simulink model "controllerReference_r2019a"  (R2019a)
settings: Solver=ode23tb  StartTime=0.0  StopTime=Inf  FixedStep=.05  RelTol=1e-3  EnableMultiTasking=on
StartFcn:
  | %tic
StopFcn:
  | %toc
model workspace (MAT data in the model file):
  A_mu = 10
  B_reff = 8.386
  Cz = 7766.25
  DCT_Param : struct (value not decoded)
  DLCXref = [0 6 7 14 33.5 34 42 50 60]
  DLCYref = [0 0 -4.5 -4 -3.75 1.5 0.5 0 0]
  D_reff = 0.25826
  Downshift_Speeds = [9.5625 12.9375 16.3125 19.6875 23.0625 26.4375 29.8125 33.1875 36.5625 39.9375 43.3125 46.6875 ... (28 elements, 4x7)]
  EngRevLim = 7000
  Pedal_Positions = [0.1 0.4 0.5 0.9]
  SUS : struct (value not decoded)
  Upshift_Speeds = [12.9375 16.3125 19.6875 33 26.4375 29.8125 33.1875 52.5 39.9375 43.3125 46.6875 77.25 ... (28 elements, 4x7)]
  VEH : struct (value not decoded)
  V_o = 16.7
  V_xlow = 1
  WH : struct (value not decoded)
  a = 1.4
  alpha_max = 1.5
  alpha_min = -1.5
  b = 1.8
  c_zo = 209651
  epsilon = 0.1
  h = 0.134
  path : struct (value not decoded)
  pio = 220000
  q_Fcx = 0
  q_Fz2 = 15.4
  q_Fzy = 0
  q_reo = 0.9974
  q_sx1 = -0.007764
  q_sx10 = 0.2824
  q_sx11 = 5.349
  q_sx12 = 0
  q_sx13 = 0
  q_sx14 = 0
  q_sx2 = 1.1915
  q_sx3 = 0.013948
  q_sx4 = 4.912
  q_sx5 = 1.02
  q_sx6 = 22.83
  q_sx7 = 0.7104
  q_sx8 = -0.023393
  q_sx9 = 0.6581
  q_sy1 = 0.00702
  q_sy2 = 0
  q_sy3 = 0.001515
  q_sy4 = 8.514e-05
  q_sy5 = 0
  q_sy6 = 0
  q_sy7 = 0.9008
  q_sy8 = -0.4089
  q_v1 = 0.0007742
  q_v2 = 0.04667
  r_Bx1 = 12.531
  r_Bx2 = 9.532
  r_Bx3 = 0
  r_By1 = 10.615
  r_By2 = 7.705
  r_By3 = 3.433e-06
  r_By4 = 0
  r_Cx1 = 1.019
  r_Cy1 = 1.0585
  r_Ex1 = -0.4487
  r_Ex2 = -0.4726
  r_Ey1 = 0.3132
  r_Ey2 = 7.63e-06
  r_Hx1 = 0.0002374
  r_Hy1 = 0.011646
  r_Hy2 = 7.63e-06
  r_Vy1 = 0.05654
  r_Vy2 = 7.63e-06
  r_Vy3 = 0
  r_Vy4 = 99.9
  r_Vy5 = 2
  r_Vy6 = 15.814
  r_o = 0.3135
  vehWidth = 2
  w = 1
symbols that are objects in the model workspace (value not decoded): VEH
undefined symbols (not defined in the file): curvature, curvatures, pathPoints, speedProfile, splineParams, Steer, Ts, velocities, xDotRef, xRef, yDotRef, yRef
libraries: autolibutils x5, simulink x5, sim3dlib x4, mpcadaslib x1, autolibshared x1, vrlib x1, vehdynlibviscommon x1
(part 2 of 2)

== system controllerReference_r2019a/Environment/Ground Feedback/3D Engine ==
  Friction : Inport
  Bus Creator : BusCreator  Inputs=4
  Bus Creator2 : BusCreator  Inputs=4
  Bus Creator3 : BusCreator  Inputs=2
  Bus Selector : BusSelector  OutputSignals=HitLoc
  Data Type Conversion : DataTypeConversion
  Demux : Demux
  Demux1 : Demux
  Passenger Vehicle Ray Trace Set : sim3dlib/Vehicle Terrain Sensor  ActorTag=SimulinkVehicle1  VehExtEn=Constant  TireRadiiExt=Constant  VehCntrLngthVal=0  TireRadiiVal=0  VehRayLngth=10  LfRayLngth=20  RfRayLngth=20  LrRayLngth=20  RrRayLngth=20  VehRayOffset=0  LfRayOffset=-1  RfRayOffset=-1  LrRayOffset=-1  RrRayOffset=-1  VehEn=on  LfEn=on  RfEn=on  LrEn=on  RrEn=on  DbgEn=off  Ts=.03  aMode=2
      settings: SourceProductName=Vehicle Dynamics Blockset  SourceProductBaseCode=VE
  Rate Transition : RateTransition
  Reshape10 : Reshape  OutputDimensionality=Row vector (2-D)
  Selector1 : Selector  InputPortWidth=5  IndexOptions=Index vector (dialog)  Indices=[2:5]  OutputSizes=1
  Signal Specification : SignalSpecification  Unit=m
  Signal Specification1 : SignalSpecification  Unit=1
  Terminator1 : Terminator
  Terminator2 : Terminator
  Zend Select : Selector  NumberOfDimensions=2  InputPortWidth=3  IndexOptions=Select all,Index vector (dialog)  Indices=[1 3],3  OutputSizes=1,1
  Ground : Outport
  wires:
  Selector1/1 -> Rate Transition/1
  Zend Select/1 -> Reshape10/1
  Bus Selector/1 -> Zend Select/1  "<HitLoc>"
  Passenger Vehicle Ray Trace Set/2 -> Terminator1/1
  Passenger Vehicle Ray Trace Set/3 -> Terminator2/1
  Reshape10/1 -> Selector1/1
  Passenger Vehicle Ray Trace Set/1 -> Bus Selector/1
  Rate Transition/1 -> Data Type Conversion/1
  Demux/2 -> Bus Creator/2  "G_FR_z"
  Demux/1 -> Bus Creator/1  "G_FL_z"
  Demux/4 -> Bus Creator/4  "G_RR_z"
  Demux/3 -> Bus Creator/3  "G_RL_z"
  Signal Specification/1 -> Demux/1
  Signal Specification1/1 -> Demux1/1
  Demux1/1 -> Bus Creator2/1  "mu_FL"
  Bus Creator/1 -> Bus Creator3/1  "z"
  Demux1/3 -> Bus Creator2/3  "mu_RL"
  Demux1/4 -> Bus Creator2/4  "mu_RR"
  Demux1/2 -> Bus Creator2/2  "mu_FR"
  Bus Creator2/1 -> Bus Creator3/2  "mu"
  Bus Creator3/1 -> Ground/1
  Friction/1 -> Signal Specification1/1
  Data Type Conversion/1 -> Signal Specification/1

== system controllerReference_r2019a/Environment/Ground Feedback/Constant ==
  Friction : Inport
  Bus Creator : BusCreator  Inputs=4
  Bus Creator2 : BusCreator  Inputs=4
  Bus Creator3 : BusCreator  Inputs=2
  Constant1 : Constant  Value=zeros(4,1)
  Demux : Demux
  Demux1 : Demux
  Signal Specification : SignalSpecification  Unit=m
  Signal Specification1 : SignalSpecification  Unit=1
  Ground : Outport
  wires:
  Constant1/1 -> Signal Specification/1
  Signal Specification/1 -> Demux/1
  Demux/4 -> Bus Creator/4  "G_RR_z"
  Demux/1 -> Bus Creator/1  "G_FL_z"
  Demux/3 -> Bus Creator/3  "G_RL_z"
  Demux/2 -> Bus Creator/2  "G_FR_z"
  Bus Creator/1 -> Bus Creator3/1  "z"
  Demux1/3 -> Bus Creator2/3  "mu_RL"
  Demux1/4 -> Bus Creator2/4  "mu_RR"
  Demux1/1 -> Bus Creator2/1  "mu_FL"
  Demux1/2 -> Bus Creator2/2  "mu_FR"
  Bus Creator2/1 -> Bus Creator3/2  "mu"
  Friction/1 -> Signal Specification1/1
  Signal Specification1/1 -> Demux1/1
  Bus Creator3/1 -> Ground/1

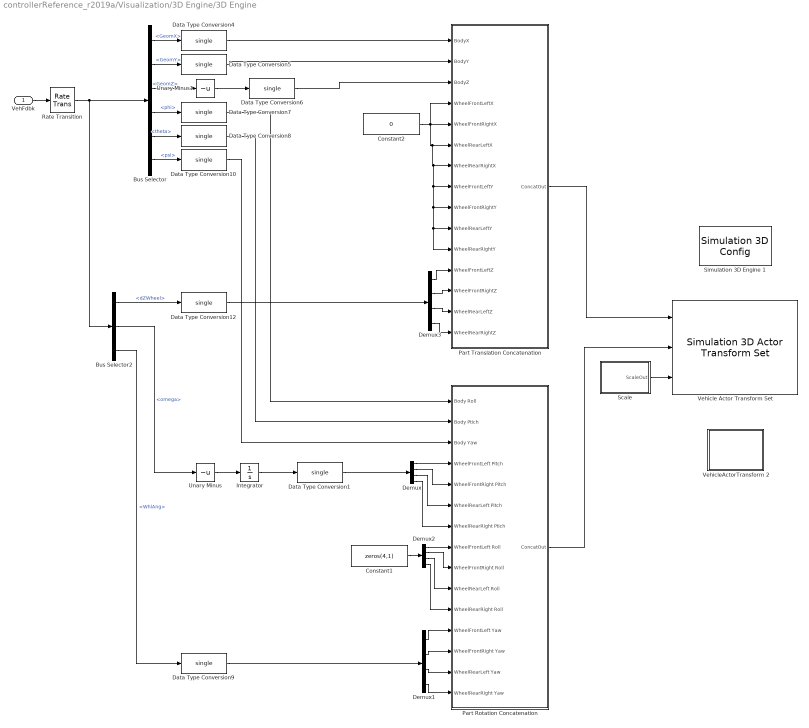
== system controllerReference_r2019a/Visualization/3D Engine/3D Engine ==
  VehFdbk : Inport
  Bus Selector : BusSelector  OutputSignals=Body.GeomX,Body.GeomY,Body.GeomZ,Body.phi,Body.theta,Body.psi
  Bus Selector2 : BusSelector  OutputSignals=Wheels.dZWheel,Wheels.omega,Driveline.WhlAng
  Constant1 : Constant  Value=zeros(4,1)  OutDataTypeStr=single
  Constant2 : Constant  Value=0  OutDataTypeStr=single
  Data Type Conversion{1,4..10,12} (9 alike) : DataTypeConversion  OutDataTypeStr=single
  Demux{,1..3} (4 alike) : Demux
  Integrator : Integrator  WrapState=on  WrappedStateUpperValue=2*pi  WrappedStateLowerValue=0  ZeroCross=off
  Part Rotation Concatenation : Subsystem
  Part Translation Concatenation : Subsystem
  Rate Transition : RateTransition  OutPortSampleTime=dt3D
  Scale : Subsystem
  Simulation 3D Engine 1 : sim3dlib/Simulation 3D Config  Priority=1  ProjectFormat=Executable  ProjectName=VehicleSimulation.exe  SceneDesc=Double lane change  OpVisEn=off  Ts=dt3D  aMode=2
      settings: AttributesFormatString=Priority: %<Priority>  SourceProductName=Vehicle Dynamics Blockset  SourceProductBaseCode=VE
  Unary Minus : UnaryMinus
  Unary Minus1 : UnaryMinus
  Vehicle Actor Transform Set : sim3dlib/Simulation 3D Actor Transform Set  ActorTag=SimulinkVehicle1  ActorType=Passenger vehicle  PassVehMesh=Muscle car  VehColor=Red  NumberOfParts=5  CustNumOfParts=3  Translation=[VEH.InitialLongPosition VEH.InitialLatPosition -VEH.InitialVertPosition; 0 0 0; 0 0 0; 0 0 0; 0 0 0]  Rotation=[VEH.InitialRollAngle VEH.InitialPitchAngle VEH.InitialYawAngle; 0 0 0; 0 0 0; 0 0 0; 0 0 0]  Scale=[1 1 1; 1 1 1; 1 1 1; 1 1 1; 1 1 1]  Ts=dt3D  aMode=2
      settings: SourceProductName=Vehicle Dynamics Blockset  SourceProductBaseCode=VE
  VehicleActorTransform 2 : Subsystem  mask{depth=-5}
      mask prompts: depth "Initital Z position, depth (m):"
  wires:
  Unary Minus1/1 -> Data Type Conversion6/1
  Unary Minus/1 -> Integrator/1
  Bus Selector2/1 -> Data Type Conversion12/1  "<dZWheel>"
  Rate Transition/1 -> Bus Selector/1, Bus Selector2/1
  Scale/1(ScaleOut) -> Vehicle Actor Transform Set/3
  Demux/4 -> Part Rotation Concatenation/7(WheelRearRight Ptich)
  Demux/3 -> Part Rotation Concatenation/6(WheelRearLeft Pitch)
  Demux/2 -> Part Rotation Concatenation/5(WheelFrontRight Pitch)
  Demux/1 -> Part Rotation Concatenation/4(WheelFrontLeft Pitch)
  Constant1/1 -> Demux2/1
  Bus Selector/4 -> Data Type Conversion7/1  "<phi>"
  Part Rotation Concatenation/1(ConcatOut) -> Vehicle Actor Transform Set/2
  Part Translation Concatenation/1(ConcatOut) -> Vehicle Actor Transform Set/1
  Data Type Conversion12/1 -> Demux3/1
  Demux3/4 -> Part Translation Concatenation/15(WheelRearRightZ)
  Demux3/3 -> Part Translation Concatenation/14(WheelRearLeftZ)
  Demux3/1 -> Part Translation Concatenation/12(WheelFrontLeftZ)
  Demux3/2 -> Part Translation Concatenation/13(WheelFrontRightZ)
  VehFdbk/1 -> Rate Transition/1
  Data Type Conversion6/1 -> Part Translation Concatenation/3(BodyZ)
  Demux1/4 -> Part Rotation Concatenation/15(WheelRearRight Yaw)
  Demux1/3 -> Part Rotation Concatenation/14(WheelRearLeft Yaw)
  Demux2/1 -> Part Rotation Concatenation/8(WheelFrontLeft Roll)
  Demux2/2 -> Part Rotation Concatenation/9(WheelFrontRight Roll)
  Demux2/3 -> Part Rotation Concatenation/10(WheelRearLeft Roll)
  Demux2/4 -> Part Rotation Concatenation/11(WheelRearRight Roll)
  Bus Selector2/3 -> Data Type Conversion9/1  "<WhlAng>"
  Bus Selector2/2 -> Unary Minus/1  "<omega>"
  Data Type Conversion9/1 -> Demux1/1
  Demux1/1 -> Part Rotation Concatenation/12(WheelFrontLeft Yaw)
  Demux1/2 -> Part Rotation Concatenation/13(WheelFrontRight Yaw)
  Integrator/1 -> Data Type Conversion1/1
  Data Type Conversion1/1 -> Demux/1
  Data Type Conversion8/1 -> Part Rotation Concatenation/2(Body Ptich)
  Data Type Conversion5/1 -> Part Translation Concatenation/2(BodyY)
  Data Type Conversion10/1 -> Part Rotation Concatenation/3(Body Yaw)
  Constant2/1 -> Part Translation Concatenation/5(WheelFrontRightX), Part Translation Concatenation/6(WheelRearLeftX), Part Translation Concatenation/7(WheelRearRightX), Part Translation Concatenation/8(WheelFrontLeftY), Part Translation Concatenation/9(WheelFrontRightY), Part Translation Concatenation/10(WheelRearLeftY), Part Translation Concatenation/11(WheelRearRightY), Part Translation Concatenation/4(WheelFrontLeftX)
  Data Type Conversion4/1 -> Part Translation Concatenation/1(BodyX)
  Data Type Conversion7/1 -> Part Rotation Concatenation/1(Body Roll)
  Bus Selector/1 -> Data Type Conversion4/1  "<GeomX>"
  Bus Selector/2 -> Data Type Conversion5/1  "<GeomY>"
  Bus Selector/3 -> Unary Minus1/1  "<GeomZ>"
  Bus Selector/6 -> Data Type Conversion10/1  "<psi>"
  Bus Selector/5 -> Data Type Conversion8/1  "<theta>"

== system controllerReference_r2019a/Visualization/3D Engine/3D Engine Disabled ==
  VehFdbk : Inport
  Terminator : Terminator
  wires:
  VehFdbk/1 -> Terminator/1

== system controllerReference_r2019a/Visualization/ISO 15037-1:2006/Disabled ==
  VehFdbk : Inport
  Cntrl : Inport  Port=2
  Terminator : Terminator
  Terminator1 : Terminator
  wires:
  Cntrl/1 -> Terminator/1
  VehFdbk/1 -> Terminator1/1

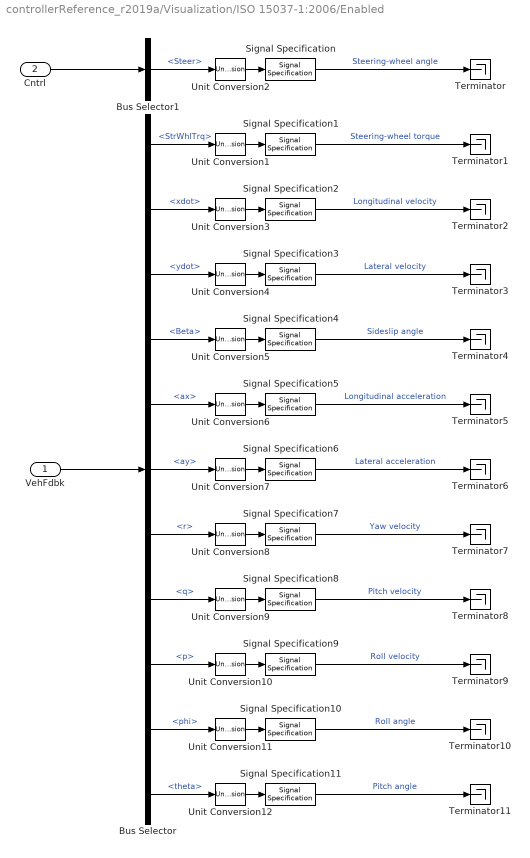
== system controllerReference_r2019a/Visualization/ISO 15037-1:2006/Enabled ==
  VehFdbk : Inport
  Cntrl : Inport  Port=2
  Bus Selector : BusSelector  OutputSignals=Steering.StrWhlTrq,Body.xdot,Body.ydot,Body.Beta,Body.ax,Body.ay,Body.r,Body.q,Body.p,Body.phi,Body.theta
  Bus Selector1 : BusSelector  OutputSignals=Steer
  Signal Specification{,4,10..11} (4 alike) : SignalSpecification  Unit=deg
  Signal Specification1 : SignalSpecification  Unit=N*m
  Signal Specification2 : SignalSpecification  Unit=km/h
  Signal Specification3 : SignalSpecification  Unit=m/s
  Signal Specification5 : SignalSpecification  Unit=m/s^2
  Signal Specification6 : SignalSpecification  Unit=m/s^2
  Signal Specification7 : SignalSpecification  Unit=deg/s
  Signal Specification8 : SignalSpecification  Unit=deg/s
  Signal Specification9 : SignalSpecification  Unit=deg/s
  Terminator{,1..11} (12 alike) : Terminator
  Unit Conversion{1..12} (12 alike) : UnitConversion
  wires:
  Bus Selector/11 -> Unit Conversion12/1  "<theta>"
  Signal Specification11/1 -> Terminator11/1  "Pitch angle"
  Unit Conversion12/1 -> Signal Specification11/1
  Bus Selector/10 -> Unit Conversion11/1  "<phi>"
  Unit Conversion11/1 -> Signal Specification10/1
  Signal Specification10/1 -> Terminator10/1  "Roll angle"
  Bus Selector/9 -> Unit Conversion10/1  "<p>"
  Signal Specification9/1 -> Terminator9/1  "Roll velocity"
  Unit Conversion10/1 -> Signal Specification9/1
  Bus Selector/8 -> Unit Conversion9/1  "<q>"
  Unit Conversion9/1 -> Signal Specification8/1
  Signal Specification8/1 -> Terminator8/1  "Pitch velocity"
  Bus Selector/7 -> Unit Conversion8/1  "<r>"
  Signal Specification7/1 -> Terminator7/1  "Yaw velocity"
  Unit Conversion8/1 -> Signal Specification7/1
  Bus Selector/6 -> Unit Conversion7/1  "<ay>"
  Unit Conversion7/1 -> Signal Specification6/1
  Signal Specification6/1 -> Terminator6/1  "Lateral acceleration"
  Bus Selector/5 -> Unit Conversion6/1  "<ax>"
  Signal Specification5/1 -> Terminator5/1  "Longitudinal acceleration"
  Unit Conversion6/1 -> Signal Specification5/1
  Bus Selector/4 -> Unit Conversion5/1  "<Beta>"
  Unit Conversion5/1 -> Signal Specification4/1
  Signal Specification4/1 -> Terminator4/1  "Sideslip angle"
  Bus Selector/3 -> Unit Conversion4/1  "<ydot>"
  Signal Specification3/1 -> Terminator3/1  "Lateral velocity"
  Unit Conversion4/1 -> Signal Specification3/1
  Bus Selector/2 -> Unit Conversion3/1  "<xdot>"
  Unit Conversion3/1 -> Signal Specification2/1
  Signal Specification2/1 -> Terminator2/1  "Longitudinal velocity"
  Signal Specification1/1 -> Terminator1/1  "Steering-wheel torque"
  Unit Conversion1/1 -> Signal Specification1/1
  Bus Selector/1 -> Unit Conversion1/1  "<StrWhlTrq>"
  Signal Specification/1 -> Terminator/1  "Steering-wheel angle"
  Unit Conversion2/1 -> Signal Specification/1
  Bus Selector1/1 -> Unit Conversion2/1  "<Steer>"
  Cntrl/1 -> Bus Selector1/1
  VehFdbk/1 -> Bus Selector/1

== system controllerReference_r2019a/Controllers/Brake Controller/Brake Pressure Control/Bang Bang ABS ==
  Pref : Inport
  xdot : Inport  Port=2
  <Kappa> : Inport  Port=3
  Abs : Abs
  Add : Sum  Inputs=-+
  Bang-bang controller : Subsystem  mask(Sign){}
      mask help: y = sign(x)
      mask Help: Sign Function:\n\t\t\ty = 1 if x > 0\n\t\t\ty = 0 if x = 0\n\t\t\ty = -1 if x < 0
      mask Display: plot(-50,-50,50,50,[-50,50],[0,0],[0,0],[-50,50],[-40,0],[-30,-30],[0,40],[30,30])
  Compare To Constant : simulink/Logic and Bit Operations/Compare To Constant  relop=>=  const=.2  OutDataTypeStr=boolean
  Compare To Constant1 : simulink/Logic and Bit Operations/Compare To Constant  relop=>=  const=.75  OutDataTypeStr=boolean
  Compare To Constant2 : simulink/Logic and Bit Operations/Compare To Constant  relop=>=  const=.5  OutDataTypeStr=boolean
  Constant : Constant  Value=.25
  Debounce : autolibutils/Debounce  DbcOn_Cnts=.1*.001  DbcOff_Cnts=.1*.001  aMode=aMode
      settings: SourceProductName=Powertrain Blockset  SourceProductBaseCode=PW
  Gain : Gain  Gain=200
  Logical Operator : Logic  Inputs=3  AllPortsSameDT=off  OutDataTypeStr=boolean
  Rate Transition : RateTransition  Deterministic=off  OutPortSampleTime=.001
  Rate Transition1 : RateTransition  Deterministic=off
  Switch : Switch  Criteria=u2 > Threshold  ZeroCross=off
  PCmd : Outport
  wires:
  Bang-bang controller/1(out_1) -> Gain/1
  Add/1 -> Bang-bang controller/1(in_1)
  Rate Transition1/1 -> PCmd/1
  <Kappa>/1 -> Rate Transition/1
  Pref/1 -> Switch/3, Compare To Constant1/1  "Pref"
  Constant/1 -> Add/2  "slip ref"
  Switch/1 -> Rate Transition1/1
  Rate Transition/1 -> Add/1, Compare To Constant/1
  Logical Operator/1 -> Debounce/1
  Compare To Constant/1 -> Logical Operator/2
  Compare To Constant1/1 -> Logical Operator/3
  Debounce/1 -> Switch/2
  xdot/1 -> Abs/1
  Abs/1 -> Compare To Constant2/1
  Compare To Constant2/1 -> Logical Operator/1
  Gain/1 -> Switch/1

== system controllerReference_r2019a/Controllers/Brake Controller/Brake Pressure Control/Open Loop ==
  Pref : Inport
  PCmd : Outport
  wires:
  Pref/1 -> PCmd/1  "Reference Slip"

== system controllerReference_r2019a/Controllers/Transmission Controller/Transmission Controller/TCM ==
  AccCmd : Inport
  EngSpd : Inport  Port=2
  VehSpdFdbk : Inport  Port=3
  function : TriggerPort  TriggerType=function-call  VariantControl=Variant
  Neutral Select : Subsystem
  Prop Shaft Speed LPF : DiscreteTransferFcn  Numerator=[0.000000000000000 0.009950166250832 ]  Denominator=[1.000000000000000 -0.990049833749168 ]  mask(DiscretizedDiscreteTransferFcn){}
      mask init:
      | %zoh
  TCM Shift Controller : Stateflow chart  TreatAsAtomicUnit=on
  prop speed to vehicle speed : Gain  Gain=0.45
  Gear Select : Outport
  wires:
  VehSpdFdbk/1 -> Prop Shaft Speed LPF/1
  TCM Shift Controller/1(GearState) -> Gear Select/1  "GearCmd"
  AccCmd/1 -> Neutral Select/1(AccCmd), TCM Shift Controller/2(pedal)  "AccCmd"
  Neutral Select/1(Neutral Select) -> TCM Shift Controller/3(Neutral)
  EngSpd/1 -> Neutral Select/2(EngSpd)
  prop speed to vehicle speed/1 -> TCM Shift Controller/1(speed)
  Prop Shaft Speed LPF/1 -> prop speed to vehicle speed/1

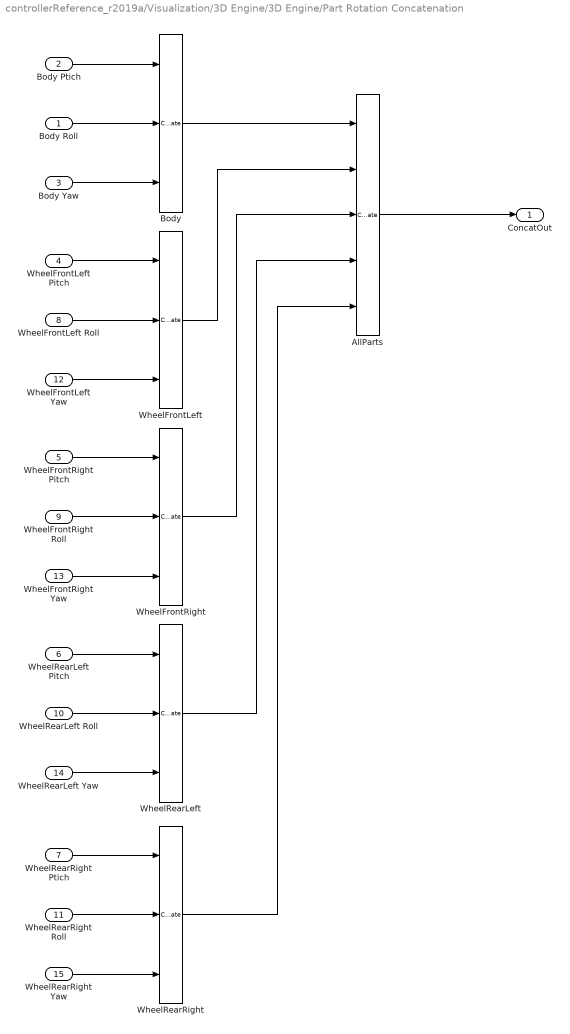
== system controllerReference_r2019a/Visualization/3D Engine/3D Engine/Part Rotation Concatenation ==
  Body Roll : Inport
  Body Ptich : Inport  Port=2
  Body Yaw : Inport  Port=3
  WheelFrontLeft Pitch : Inport  Port=4
  WheelFrontRight Pitch : Inport  Port=5
  WheelRearLeft Pitch : Inport  Port=6
  WheelRearRight Ptich : Inport  Port=7
  WheelFrontLeft Roll : Inport  Port=8
  WheelFrontRight Roll : Inport  Port=9
  WheelRearLeft Roll : Inport  Port=10
  WheelRearRight Roll : Inport  Port=11
  WheelFrontLeft Yaw : Inport  Port=12
  WheelFrontRight Yaw : Inport  Port=13
  WheelRearLeft Yaw : Inport  Port=14
  WheelRearRight Yaw : Inport  Port=15
  AllParts : Concatenate  NumInputs=5  Mode=Multidimensional array
  Body : Concatenate  NumInputs=3  Mode=Multidimensional array  ConcatenateDimension=2
  WheelFrontLeft : Concatenate  NumInputs=3  Mode=Multidimensional array  ConcatenateDimension=2
  WheelFrontRight : Concatenate  NumInputs=3  Mode=Multidimensional array  ConcatenateDimension=2
  WheelRearLeft : Concatenate  NumInputs=3  Mode=Multidimensional array  ConcatenateDimension=2
  WheelRearRight : Concatenate  NumInputs=3  Mode=Multidimensional array  ConcatenateDimension=2
  ConcatOut : Outport
  wires:
  Body Ptich/1 -> Body/1
  Body Yaw/1 -> Body/3
  WheelFrontLeft Pitch/1 -> WheelFrontLeft/1
  WheelFrontLeft Yaw/1 -> WheelFrontLeft/3
  WheelFrontLeft Roll/1 -> WheelFrontLeft/2
  Body Roll/1 -> Body/2
  WheelFrontLeft/1 -> AllParts/2
  WheelRearRight Ptich/1 -> WheelRearRight/1
  Body/1 -> AllParts/1
  WheelRearLeft/1 -> AllParts/4
  WheelFrontRight/1 -> AllParts/3
  WheelRearRight Yaw/1 -> WheelRearRight/3
  WheelFrontRight Roll/1 -> WheelFrontRight/2
  WheelFrontRight Pitch/1 -> WheelFrontRight/1
  WheelRearRight Roll/1 -> WheelRearRight/2
  WheelRearLeft Yaw/1 -> WheelRearLeft/3
  AllParts/1 -> ConcatOut/1
  WheelRearLeft Roll/1 -> WheelRearLeft/2
  WheelRearRight/1 -> AllParts/5
  WheelRearLeft Pitch/1 -> WheelRearLeft/1
  WheelFrontRight Yaw/1 -> WheelFrontRight/3

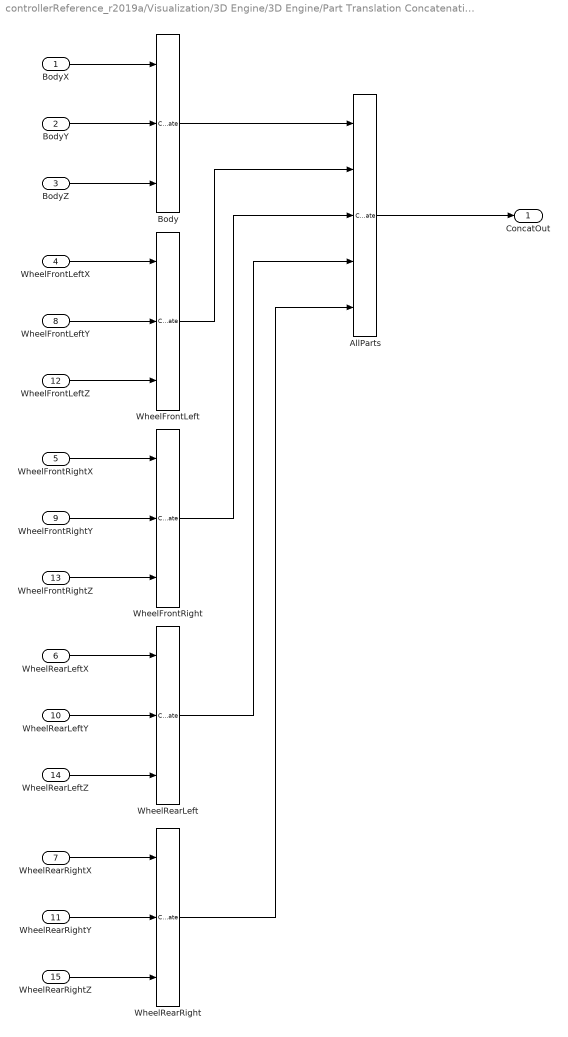
== system controllerReference_r2019a/Visualization/3D Engine/3D Engine/Part Translation Concatenation ==
  BodyX : Inport
  BodyY : Inport  Port=2
  BodyZ : Inport  Port=3
  WheelFrontLeftX : Inport  Port=4
  WheelFrontRightX : Inport  Port=5
  WheelRearLeftX : Inport  Port=6
  WheelRearRightX : Inport  Port=7
  WheelFrontLeftY : Inport  Port=8
  WheelFrontRightY : Inport  Port=9
  WheelRearLeftY : Inport  Port=10
  WheelRearRightY : Inport  Port=11
  WheelFrontLeftZ : Inport  Port=12
  WheelFrontRightZ : Inport  Port=13
  WheelRearLeftZ : Inport  Port=14
  WheelRearRightZ : Inport  Port=15
  AllParts : Concatenate  NumInputs=5  Mode=Multidimensional array
  Body : Concatenate  NumInputs=3  Mode=Multidimensional array  ConcatenateDimension=2
  WheelFrontLeft : Concatenate  NumInputs=3  Mode=Multidimensional array  ConcatenateDimension=2
  WheelFrontRight : Concatenate  NumInputs=3  Mode=Multidimensional array  ConcatenateDimension=2
  WheelRearLeft : Concatenate  NumInputs=3  Mode=Multidimensional array  ConcatenateDimension=2
  WheelRearRight : Concatenate  NumInputs=3  Mode=Multidimensional array  ConcatenateDimension=2
  ConcatOut : Outport
  wires:
  BodyX/1 -> Body/1
  BodyZ/1 -> Body/3
  WheelFrontLeftX/1 -> WheelFrontLeft/1
  WheelFrontLeftZ/1 -> WheelFrontLeft/3
  WheelFrontLeftY/1 -> WheelFrontLeft/2
  BodyY/1 -> Body/2
  WheelFrontLeft/1 -> AllParts/2
  WheelRearRightX/1 -> WheelRearRight/1
  Body/1 -> AllParts/1
  WheelRearLeft/1 -> AllParts/4
  WheelFrontRight/1 -> AllParts/3
  WheelRearRightZ/1 -> WheelRearRight/3
  WheelFrontRightY/1 -> WheelFrontRight/2
  WheelFrontRightX/1 -> WheelFrontRight/1
  WheelRearRightY/1 -> WheelRearRight/2
  WheelRearLeftZ/1 -> WheelRearLeft/3
  AllParts/1 -> ConcatOut/1
  WheelRearLeftY/1 -> WheelRearLeft/2
  WheelRearRight/1 -> AllParts/5
  WheelRearLeftX/1 -> WheelRearLeft/1
  WheelFrontRightZ/1 -> WheelFrontRight/3

== system controllerReference_r2019a/Visualization/3D Engine/3D Engine/Scale ==
  Constant{1..12,17,32..33} (15 alike) : Constant  OutDataTypeStr=single
  PartConcatenation : Subsystem
  ScaleOut : Outport
  wires:
  Constant10/1 -> PartConcatenation/15(WheelRearRightZ)
  Constant9/1 -> PartConcatenation/14(WheelRearRightY)
  Constant11/1 -> PartConcatenation/13(WheelRearRightX)
  Constant7/1 -> PartConcatenation/12(WheelRearLeftZ)
  Constant6/1 -> PartConcatenation/11(WheelRearLeftY)
  Constant8/1 -> PartConcatenation/10(WheelRearLeftX)
  Constant4/1 -> PartConcatenation/9(WheelFrontRightZ)
  Constant3/1 -> PartConcatenation/8(WheelFrontRightY)
  Constant5/1 -> PartConcatenation/7(WheelFrontRightX)
  Constant2/1 -> PartConcatenation/6(WheelFrontLeftZ)
  Constant1/1 -> PartConcatenation/5(WheelFrontLeftY)
  Constant33/1 -> PartConcatenation/4(WheelFrontLeftX)
  Constant32/1 -> PartConcatenation/3(BodyZ)
  Constant17/1 -> PartConcatenation/2(BodyY)
  Constant12/1 -> PartConcatenation/1(BodyX)
  PartConcatenation/1(ConcatOut) -> ScaleOut/1

== system controllerReference_r2019a/Visualization/3D Engine/3D Engine/VehicleActorTransform 2 ==
  Constant : Constant  Value=[0 0 depth; 0 0 0; 0 0 0; 0 0 0; 0 0 0]
  Constant1 : Constant  Value=[0 0 0; 0 0 0; 0 0 0; 0 0 0; 0 0 0]
  Constant2 : Constant  Value=ones(5,3)
  Vehicle Actor Transform Set1 : sim3dlib/Simulation 3D Actor Transform Set  ActorTag=SimulinkVehicle2  ActorType=Passenger vehicle  PassVehMesh=Muscle car  VehColor=Green  NumberOfParts=5  CustNumOfParts=3  Translation=[0 0 depth; 0 0 0; 0 0 0; 0 0 0; 0 0 0]  Rotation=[0 0 0; 0 0 0; 0 0 0; 0 0 0; 0 0 0]  Scale=[1 1 1; 1 1 1; 1 1 1; 1 1 1; 1 1 1]  Ts=-1  aMode=aMode
      settings: SourceProductName=Vehicle Dynamics Blockset  SourceProductBaseCode=VE
  wires:
  Constant/1 -> Vehicle Actor Transform Set1/1
  Constant2/1 -> Vehicle Actor Transform Set1/3
  Constant1/1 -> Vehicle Actor Transform Set1/2

== system controllerReference_r2019a/Controllers/Brake Controller/Brake Pressure Control/Bang Bang ABS/Bang-bang controller ==
  in_1 : Inport
  Constant : Constant  Value=0
  Data Type Conversion1 : DataTypeConversion  OutDataTypeStr=double  SaturateOnIntegerOverflow=on  RndMeth=Zero
  Data Type Conversion2 : DataTypeConversion  OutDataTypeStr=double  SaturateOnIntegerOverflow=on  RndMeth=Zero
  Relational Operator : RelationalOperator  Operator=>  OutDataTypeStr=boolean  RndMeth=Nearest  InputSameDT=on
  Relational Operator1 : RelationalOperator  Operator=<  OutDataTypeStr=boolean  RndMeth=Nearest  InputSameDT=on
  Sum : Sum  Inputs=+-  SaturateOnIntegerOverflow=on  InputSameDT=on  OutDataTypeStr=Inherit: Same as first input
  out_1 : Outport  InitialOutput=0
  wires:
  Data Type Conversion2/1 -> Sum/2
  Data Type Conversion1/1 -> Sum/1
  Sum/1 -> out_1/1
  Relational Operator/1 -> Data Type Conversion1/1
  Relational Operator1/1 -> Data Type Conversion2/1
  Constant/1 -> Relational Operator/2, Relational Operator1/2
  in_1/1 -> Relational Operator1/1, Relational Operator/1

== system controllerReference_r2019a/Controllers/Transmission Controller/Transmission Controller/TCM/Neutral Select ==
  AccCmd : Inport
  EngSpd : Inport  Port=2
  Constant : Constant  Value=1200
  Constant1 : Constant  Value=1e-6
  Logical Operator : Logic  AllPortsSameDT=off  OutDataTypeStr=boolean
  Relational Operator : RelationalOperator  Operator=<=  OutDataTypeStr=boolean  RndMeth=Simplest
  Relational Operator1 : RelationalOperator  Operator=<=  OutDataTypeStr=boolean  RndMeth=Simplest
  Neutral Select : Outport
  wires:
  EngSpd/1 -> Relational Operator/1
  Relational Operator1/1 -> Logical Operator/1
  AccCmd/1 -> Relational Operator1/1
  Constant1/1 -> Relational Operator1/2
  Logical Operator/1 -> Neutral Select/1
  Constant/1 -> Relational Operator/2
  Relational Operator/1 -> Logical Operator/2

== system controllerReference_r2019a/Controllers/Transmission Controller/Transmission Controller/TCM/TCM Shift Controller/calc ==
  note: Determine if next gear will be
      | higher or lower than current gear
  gear : Inport
  pedal : Inport  Port=2
  speed : Inport  Port=3
  f : TriggerPort  TriggerType=function-call  VariantControl=Variant  StatesWhenEnabling=reset
      settings: CopyFcn=Stateflow.SLINSF.SimulinkMan.removeBlockPreDeleteFcn  PreDeleteFcn=Stateflow.SLINSF.SimulinkMan.unsafePredeleteFcn
  Add1 : Sum  Inputs=+-
  Add3 : Sum  Inputs=+-
  Add4 : Sum  Inputs=+-
  Calculate Upshift Threshold : Lookup_n-D  BreakpointsForDimension1=Pedal_Positions  BreakpointsForDimension2=1:7  Table=Upshift_Speeds  ExtrapMethod=Clip  UseLastTableValue=on  InternalRulePriority=Speed  RndMeth=Simplest  InputSameDT=on
  Calculate Downshift Threshold : Lookup_n-D  BreakpointsForDimension1=Pedal_Positions  BreakpointsForDimension2=2:8  Table=Downshift_Speeds  ExtrapMethod=Clip  UseLastTableValue=on  InternalRulePriority=Speed  RndMeth=Simplest  InputSameDT=on
  SpdThr : Outport
  wires:
  pedal/1 -> Calculate Downshift Threshold/1, Calculate Upshift Threshold/1
  gear/1 -> Calculate Downshift Threshold/2, Calculate Upshift Threshold/2
  Calculate Downshift Threshold/1 -> Add3/2
  Calculate Upshift Threshold/1 -> Add1/1
  speed/1 -> Add1/2, Add3/1
  Add1/1 -> Add4/1
  Add3/1 -> Add4/2
  Add4/1 -> SpdThr/1

== system controllerReference_r2019a/Controllers/Transmission Controller/Transmission Controller/TCM/TCM Shift Controller/calc_down ==
  gear : Inport
  pedal : Inport  Port=2
  f : TriggerPort  TriggerType=function-call  VariantControl=Variant  StatesWhenEnabling=reset
      settings: CopyFcn=Stateflow.SLINSF.SimulinkMan.removeBlockPreDeleteFcn  PreDeleteFcn=Stateflow.SLINSF.SimulinkMan.unsafePredeleteFcn
  Calculate Downshift Threshold : Lookup_n-D  BreakpointsForDimension1=Pedal_Positions  BreakpointsForDimension2=2:8  Table=Downshift_Speeds  ExtrapMethod=Clip  UseLastTableValue=on  InternalRulePriority=Speed  RndMeth=Simplest  InputSameDT=on
  down_th : Outport
  wires:
  Calculate Downshift Threshold/1 -> down_th/1
  gear/1 -> Calculate Downshift Threshold/2
  pedal/1 -> Calculate Downshift Threshold/1

== system controllerReference_r2019a/Controllers/Transmission Controller/Transmission Controller/TCM/TCM Shift Controller/calc_up ==
  gear : Inport
  pedal : Inport  Port=2
  f : TriggerPort  TriggerType=function-call  VariantControl=Variant  StatesWhenEnabling=reset
      settings: CopyFcn=Stateflow.SLINSF.SimulinkMan.removeBlockPreDeleteFcn  PreDeleteFcn=Stateflow.SLINSF.SimulinkMan.unsafePredeleteFcn
  Calculate Upshift Threshold : Lookup_n-D  BreakpointsForDimension1=Pedal_Positions  BreakpointsForDimension2=1:7  Table=Upshift_Speeds  ExtrapMethod=Clip  UseLastTableValue=on  InternalRulePriority=Speed  RndMeth=Simplest  InputSameDT=on
  up_th : Outport
  wires:
  Calculate Upshift Threshold/1 -> up_th/1
  pedal/1 -> Calculate Upshift Threshold/1
  gear/1 -> Calculate Upshift Threshold/2

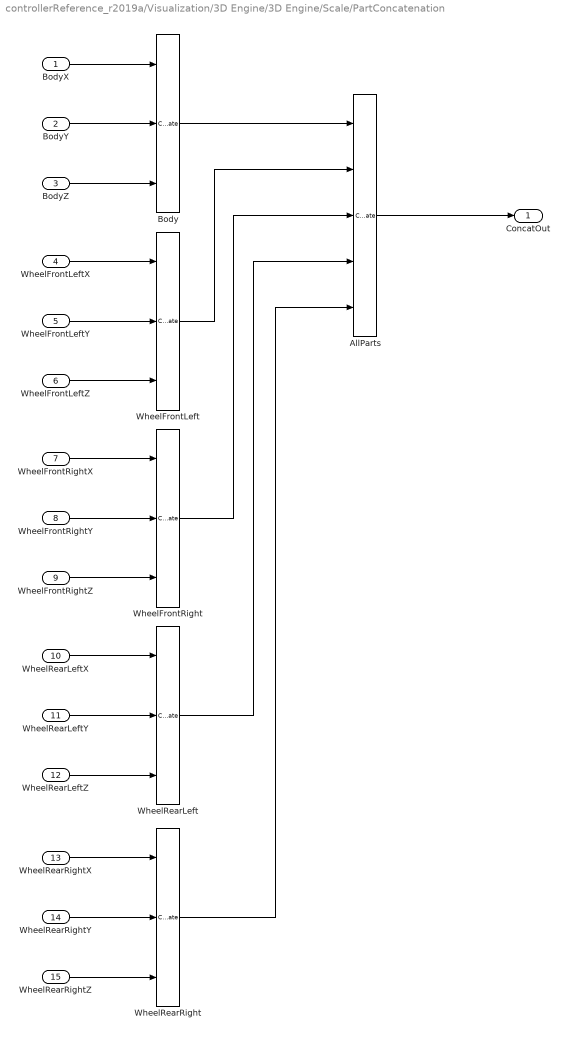
== system controllerReference_r2019a/Visualization/3D Engine/3D Engine/Scale/PartConcatenation ==
  BodyX : Inport
  BodyY : Inport  Port=2
  BodyZ : Inport  Port=3
  WheelFrontLeftX : Inport  Port=4
  WheelFrontLeftY : Inport  Port=5
  WheelFrontLeftZ : Inport  Port=6
  WheelFrontRightX : Inport  Port=7
  WheelFrontRightY : Inport  Port=8
  WheelFrontRightZ : Inport  Port=9
  WheelRearLeftX : Inport  Port=10
  WheelRearLeftY : Inport  Port=11
  WheelRearLeftZ : Inport  Port=12
  WheelRearRightX : Inport  Port=13
  WheelRearRightY : Inport  Port=14
  WheelRearRightZ : Inport  Port=15
  AllParts : Concatenate  NumInputs=5  Mode=Multidimensional array
  Body : Concatenate  NumInputs=3  Mode=Multidimensional array  ConcatenateDimension=2
  WheelFrontLeft : Concatenate  NumInputs=3  Mode=Multidimensional array  ConcatenateDimension=2
  WheelFrontRight : Concatenate  NumInputs=3  Mode=Multidimensional array  ConcatenateDimension=2
  WheelRearLeft : Concatenate  NumInputs=3  Mode=Multidimensional array  ConcatenateDimension=2
  WheelRearRight : Concatenate  NumInputs=3  Mode=Multidimensional array  ConcatenateDimension=2
  ConcatOut : Outport
  wires:
  BodyX/1 -> Body/1
  BodyZ/1 -> Body/3
  WheelFrontLeftX/1 -> WheelFrontLeft/1
  WheelFrontLeftZ/1 -> WheelFrontLeft/3
  WheelFrontLeftY/1 -> WheelFrontLeft/2
  BodyY/1 -> Body/2
  WheelFrontLeft/1 -> AllParts/2
  WheelRearRightX/1 -> WheelRearRight/1
  Body/1 -> AllParts/1
  WheelRearLeft/1 -> AllParts/4
  WheelFrontRight/1 -> AllParts/3
  WheelRearRightZ/1 -> WheelRearRight/3
  WheelFrontRightY/1 -> WheelFrontRight/2
  WheelFrontRightX/1 -> WheelFrontRight/1
  WheelRearRightY/1 -> WheelRearRight/2
  WheelRearLeftZ/1 -> WheelRearLeft/3
  AllParts/1 -> ConcatOut/1
  WheelRearLeftY/1 -> WheelRearLeft/2
  WheelRearRight/1 -> AllParts/5
  WheelRearLeftX/1 -> WheelRearLeft/1
  WheelFrontRightZ/1 -> WheelFrontRight/3

== stateflow chart controllerReference_r2019a/Controllers/Transmission Controller/Transmission Controller/TCM/TCM Shift Controller ==
  settings: sampleTime=0.01
  state GearState [parallel]
    settings: executionOrder=1
    state Neutral
      en:
      GearState = 0;
    state G1
      en:
      GearState = 1;
    state G2
      en:
      GearState = 2;
      du:
      [SpdThr] = calc(2,pedal,speed);
    state G3
      en:
      GearState = 3;
      du:
      [SpdThr] = calc(3,pedal,speed);
    state G8
      en:
      GearState = 8;
    state G7
      en:
      GearState = 7;
    state G6
      en:
      GearState = 6;
    state G5
      en:GearState=5;
      du:[SpdThr]=calc(5,pedal,speed);
    state G4
      en:
      GearState = 4;
      du:
      [SpdThr] = calc(4,pedal,speed);
    (default) -> G1
    Neutral -> G1 : [~Neutral]
    G1 -> G2 [order 1] : Up
    G2 -> G3 [order 1] : Up
    G1 -> Neutral [order 2] : [Neutral]
    G2 -> G1 [order 2] : Down
    G3 -> G2 [order 2] : Down
    G3 -> G4 [order 1] : Up
    G4 -> G3 [order 2] : Down
    G7 -> G8 [order 1] : Up
    G5 -> G6 [order 1] : Up
    G6 -> G7 [order 1] : Up
    G4 -> G5 [order 1] : Up
    G5 -> G4 [order 2] : Down
    G6 -> G5 [order 2] : Down
    G7 -> G6 [order 2] : Down
    G8 -> G7 : Down
  state SelectionState [parallel]
    du:[up_th]=calc_up(GearState,pedal);
    du:[down_th]=calc_down(GearState,pedal);
    settings: executionOrder=2
    state SteadyState
      en:
      clutchControl = 0;
    state preDownShifting
    state preUpShifting
    state UpShifting
      en:
      GearState = GearState + 0.5;
    state DownShifting
      en:
      GearState = GearState - 0.5;
    (default) -> SteadyState
    SteadyState -> (junction 62) [order 1] : [speed < down_th && ...
        | GearState >1]
    SteadyState -> (junction 128) [order 2] : [speed > up_th &&...
        | GearState <= 5 && ...
        | floor(GearState) == GearState]
    (junction 62) -> preDownShifting
    (junction 128) -> preUpShifting
    (junction 168) -> SteadyState
    (junction 23) -> SteadyState
    (junction 161) -> SteadyState
    preDownShifting -> (junction 168) [order 2] : [speed >= down_th]
    preUpShifting -> (junction 161) [order 2] : [speed <= up_th]
    preUpShifting -> UpShifting [order 1] : after(0.5,sec)
        | [speed>up_th]
    preDownShifting -> DownShifting [order 1] : after(0.5, sec)
        | [speed < down_th - 2]
    DownShifting -> (junction 23) : {GearState.Down;}
    UpShifting -> (junction 23) : {GearState.Up;}
  state up_th = calc_up(gear,pedal) [function]
  state down_th = calc_down(gear,pedal) [function]
  state SpdThr = calc(gear,pedal,speed) [function]
  data: gear function_input; pedal function_input; up_th function_output; gear function_input; pedal function_input; down_th function_output; gear function_input; pedal function_input; SpdThr function_output; speed function_input; GearState output int8; speed input; pedal input; clutchControl local double; SpdThr local double; Neutral input; up_th local double; down_th local double
  events: Up local EITHER_EDGE_EVENT; Down local EITHER_EDGE_EVENT

== matlab function controllerReference_r2019a/Subsystem/controllerReference ==
  data: xRef output; yRef output; xDotRef output; vehicleX input; yDotRef output; vehicleY input; pathPoints input; splineParams input; velocities input; curvatures input; curvature output
function [xRef, yRef, xDotRef, yDotRef, curvature] = controllerReference(vehicleX, vehicleY, pathPoints, splineParams, velocities, curvatures)
    % [lateralReference, referenceVelocity] = controllerReference(vehiclePosition, vehicleHeading, evaluator, splx, sply)
    
    
    % Hold the hand of Simulink and tell it what types to expect
    xRef                = 0;
    yRef                = 0;
    xDotRef             = 0;
    yDotRef             = 0;
    
    % Find closest point to the vehicle position on the spline
    d = ones(length(pathPoints),1) * [vehicleX, vehicleY] - pathPoints;
    d = vecnorm(d');
    [minVal,minIndex]   = min(d);
    
    xRef                = pathPoints(minIndex,1);
    yRef                = pathPoints(minIndex,2);
    
    curvature           = curvatures(minIndex);
    
    % Reference velocity
    referenceVelocity   = velocities(minIndex);
    if minIndex<length(pathPoints)
        tangent = pathPoints(minIndex+1,:)-pathPoints(minIndex,:);
    else
        tangent = pathPoints(minIndex,:)-pathPoints(minIndex-1,:);
    end
    tangent             = tangent / norm(tangent);
    
    xDotRef             = referenceVelocity*tangent(1);
    yDotRef             = referenceVelocity*tangent(2);
    

end
